simulink model "progetto_condizionatore_controllore"  (R2022a)
settings: Solver=VariableStepAuto  StartTime=0.0  StopTime=5*ta  RelTol=1e-3
values from neighbouring files (symbols this model uses):
  A = [(-gamma_cs/C_c) (gamma_cs/C_c); (gamma_cs/C_s) -((gamma_cs/C_s)+(gamma_sa/C_s))]    [Progetto_condizionatore.m]
  B = [1/C_c; 0]    [Progetto_condizionatore.m]
  C = [0 1]    [Progetto_condizionatore.m]
  C_s = 45225    [Progetto_condizionatore.m]
  gamma_sa = 2.3    [Progetto_condizionatore.m]
  K = place (A,B, auto_desiderati)    [Progetto_condizionatore.m]
  kr = -1/(C*((A-B*K)\B))    [Progetto_condizionatore.m]
  M = M'    [Progetto_condizionatore.m]
  temp_amb = 30    [Progetto_condizionatore.m]
  temp_des = 20    [Progetto_condizionatore.m]
  x0 = [23; 25]    [Progetto_condizionatore.m]
settings Model: Creator=Mattia  LastModifiedBy=Mattia

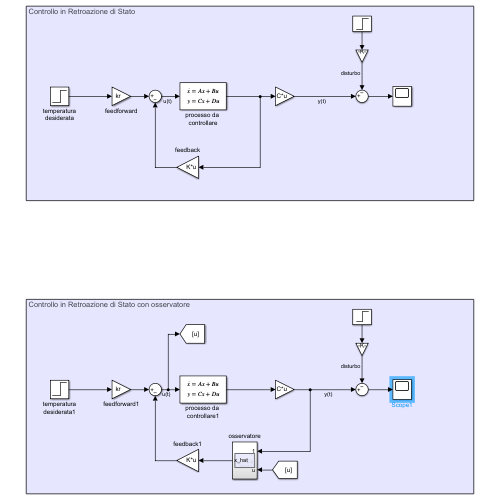
[thumbnail: Simulink's stored preview of the top-level diagram]
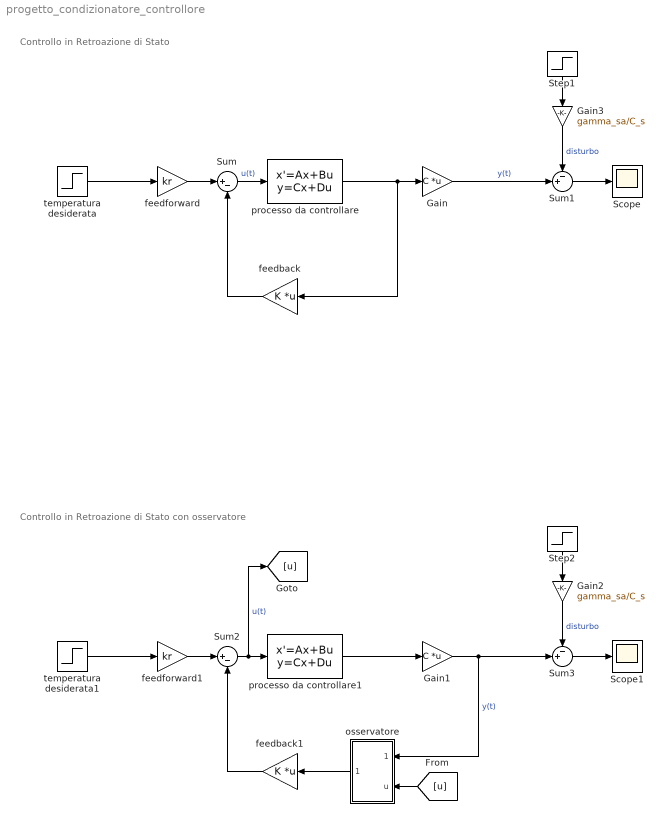
== system progetto_condizionatore_controllore ==
  note: Controllo in Retroazione di Stato
  note: Controllo in Retroazione di Stato con osservatore
  Gain : Gain  Gain=C  Multiplication=Matrix(K*u)
  Gain1 : Gain  Gain=C  Multiplication=Matrix(K*u)
  Gain2 : Gain  Gain=gamma_sa/C_s
  Gain3 : Gain  Gain=gamma_sa/C_s
  Scope : Scope
  Scope1 : Scope
  Step1 : Step  Time=0  After=temp_amb  SampleTime=0
  Step2 : Step  Time=0  After=temp_amb  SampleTime=0
  Sum : Sum  Inputs=|+-
  Sum1 : Sum  Inputs=-+|
  Sum2 : Sum  Inputs=|+-
  Sum3 : Sum  Inputs=-+|
  feedback : Gain  Gain=K  Multiplication=Matrix(K*u)
  feedback1 : Gain  Gain=K  Multiplication=Matrix(K*u)
  feedforward : Gain  Gain=kr
  feedforward1 : Gain  Gain=kr
  osservatore : Subsystem
  processo da controllare : StateSpace  A=A  B=B  C=eye(2)  D=zeros(2,1)  InitialCondition=x0
  processo da controllare1 : StateSpace  A=A  B=B  C=eye(2)  D=zeros(2,1)  InitialCondition=x0
  temperatura desiderata : Step  Time=0  After=temp_des  SampleTime=0
  temperatura desiderata1 : Step  Time=0  After=temp_des  SampleTime=0
  wires:
  temperatura desiderata/1 -> feedforward/1
  feedforward/1 -> Sum/1
  Sum/1 -> processo da controllare/1  "u(t)"
  Gain/1 -> Sum1/2  "y(t)"
  processo da controllare/1 -> feedback/1, Gain/1
  feedback/1 -> Sum/2
  Step1/1 -> Gain3/1
  Gain3/1 -> Sum1/1  "disturbo"
  Sum1/1 -> Scope/1
  [u] -> osservatore/2(u)
  Gain1/1 -> osservatore/1(In1), Sum3/2  "y(t)"
  feedforward1/1 -> Sum2/1
  Sum2/1 -> [u], processo da controllare1/1  "u(t)"
  Gain2/1 -> Sum3/1  "disturbo"
  Step2/1 -> Gain2/1
  Sum3/1 -> Scope1/1
  temperatura desiderata1/1 -> feedforward1/1
  feedback1/1 -> Sum2/2
  processo da controllare1/1 -> Gain1/1
  osservatore/1(x_hat) -> feedback1/1

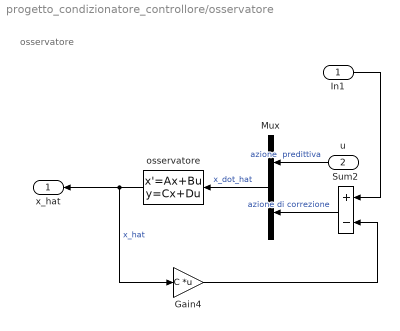
== system progetto_condizionatore_controllore/osservatore ==
  note: osservatore
  In1 : Inport
  u : Inport  Port=2
  Gain4 : Gain  Gain=C  Multiplication=Matrix(K*u)
  Mux : Mux  Inputs=2
  Sum2 : Sum  Inputs=+-
  osservatore : StateSpace  A=A  B=[B M]  C=eye(2)  D=zeros(2,2)  InitialCondition=x0
  x_hat : Outport
  wires:
  Sum2/1 -> Mux/2  "azione di correzione"
  Mux/1 -> osservatore/1  "x_dot_hat"
  In1/1 -> Sum2/1
  osservatore/1 -> x_hat/1, Gain4/1  "x_hat"
  Gain4/1 -> Sum2/2
  u/1 -> Mux/1  "azione  predittiva"
